simulink subsystem "suspensionThreeDOF"  (R2023a)
settings: Solver=VariableStepAuto  StartTime=0.0  StopTime=10.0  RelTol=1e-3
model mask{obj=obj}
  mask prompts: obj "Spring Object:"
settings Model: Creator=grouleau  LastModifiedBy=grouleau

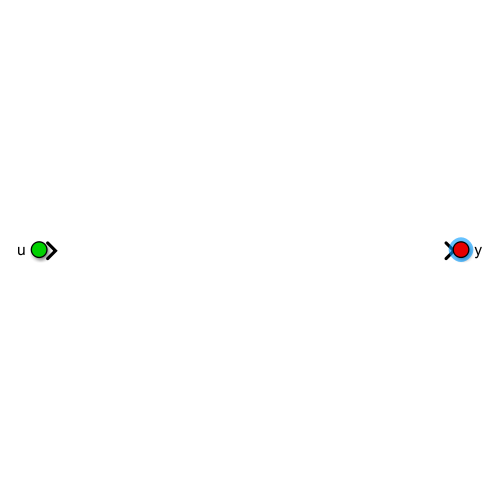
[thumbnail: Simulink's stored preview of the top-level diagram]
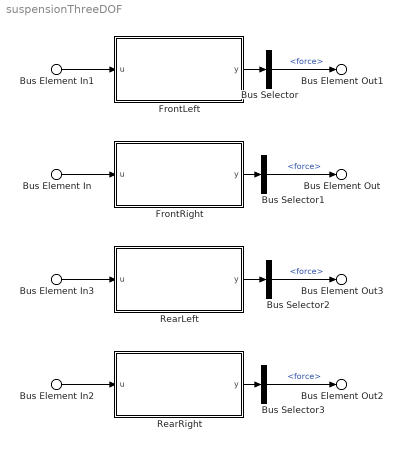
== system suspensionThreeDOF ==
  Bus Element In3 : Inport  PortName=u  Element=RearLeft
  Bus Element In1 : Inport  PortName=u  Element=FrontLeft
  Bus Element In : Inport  PortName=u  Element=FrontRight
  Bus Element In2 : Inport  PortName=u  Element=RearRight
  Bus Selector{,1..3} (4 alike) : BusSelector  OutputSignals=force
  FrontLeft : Subsystem  Variant=on  VariantChoicesSpecifier=obj.getVariantChoices()  VariantControlMode=label  LabelModeActiveChoice=suspension  mask{obj=obj.FrontLeft}
      mask prompts: obj "Part Object"
  FrontRight : Subsystem  Variant=on  VariantChoicesSpecifier=obj.getVariantChoices()  VariantControlMode=label  LabelModeActiveChoice=suspension  mask{obj=obj.FrontRight}
      mask prompts: obj "Part Object"
  RearLeft : Subsystem  Variant=on  VariantChoicesSpecifier=obj.getVariantChoices()  VariantControlMode=label  LabelModeActiveChoice=suspension  mask{obj=obj.RearLeft}
      mask prompts: obj "Part Object"
  RearRight : Subsystem  Variant=on  VariantChoicesSpecifier=obj.getVariantChoices()  VariantControlMode=label  LabelModeActiveChoice=suspension  mask{obj=obj.FrontRight}
      mask prompts: obj "Part Object"
  Bus Element Out1 : Outport  PortName=y  Element=Forces.FrontLeft
  Bus Element Out : Outport  PortName=y  Element=Forces.FrontRight
  Bus Element Out3 : Outport  PortName=y  Element=Forces.RearLeft
  Bus Element Out2 : Outport  PortName=y  Element=Forces.RearRight
  wires:
  FrontRight/1(y) -> Bus Selector1/1
  Bus Selector/1 -> Bus Element Out1/1  "<force>"
  Bus Element In/1 -> FrontRight/1(u)
  Bus Element In1/1 -> FrontLeft/1(u)
  FrontLeft/1(y) -> Bus Selector/1
  Bus Selector1/1 -> Bus Element Out/1  "<force>"
  Bus Selector3/1 -> Bus Element Out2/1  "<force>"
  RearLeft/1(y) -> Bus Selector2/1
  Bus Element In3/1 -> RearLeft/1(u)
  Bus Element In2/1 -> RearRight/1(u)
  Bus Selector2/1 -> Bus Element Out3/1  "<force>"
  RearRight/1(y) -> Bus Selector3/1

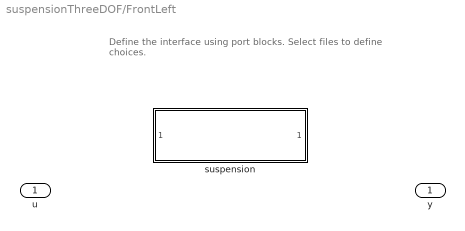
== system suspensionThreeDOF/FrontLeft ==
  note: Define the interface using port blocks.
      | Select files to define choices.
  u : Inport
  suspension : Subsystem  VariantControl=suspension  ReferencedSubsystem=suspension  obj=obj
  y : Outport

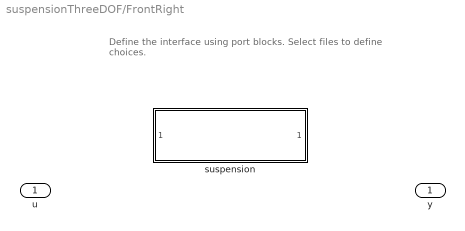
== system suspensionThreeDOF/FrontRight ==
  note: Define the interface using port blocks.
      | Select files to define choices.
  u : Inport
  suspension : Subsystem  VariantControl=suspension  ReferencedSubsystem=suspension  obj=obj
  y : Outport

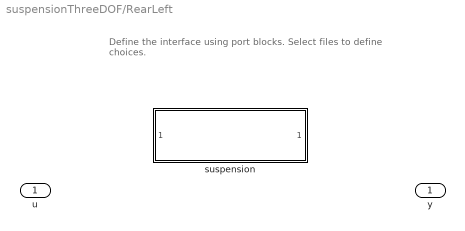
== system suspensionThreeDOF/RearLeft ==
  note: Define the interface using port blocks.
      | Select files to define choices.
  u : Inport
  suspension : Subsystem  VariantControl=suspension  ReferencedSubsystem=suspension  obj=obj
  y : Outport

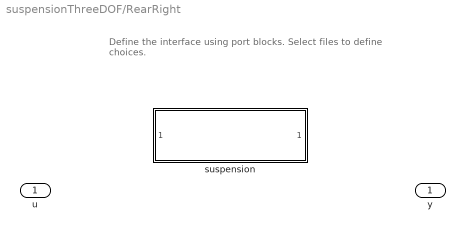
== system suspensionThreeDOF/RearRight ==
  note: Define the interface using port blocks.
      | Select files to define choices.
  u : Inport
  suspension : Subsystem  VariantControl=suspension  ReferencedSubsystem=suspension  obj=obj
  y : Outport
